simulink model "LAB9PUNKT2"  (R2022b)
settings: Solver=VariableStepAuto  StartTime=0.0  StopTime=10.0  RelTol=1e-3
settings Model: Creator=Wikor  LastModifiedBy=mateu
settings DebuggingCC: UnconnectedInputMsg=warning  UnconnectedOutputMsg=warning  UnconnectedLineMsg=warning
settings ModelReferenceCC: EnableRefExpFcnMdlSchedulingChecks=on
settings RTWCC: DLArmComputeVersion=19.05

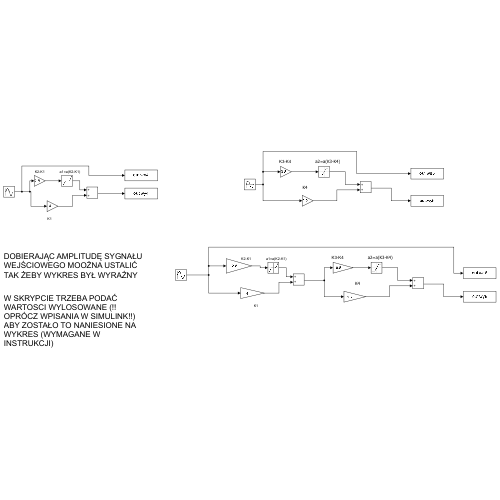
[thumbnail: Simulink's stored preview of the top-level diagram]
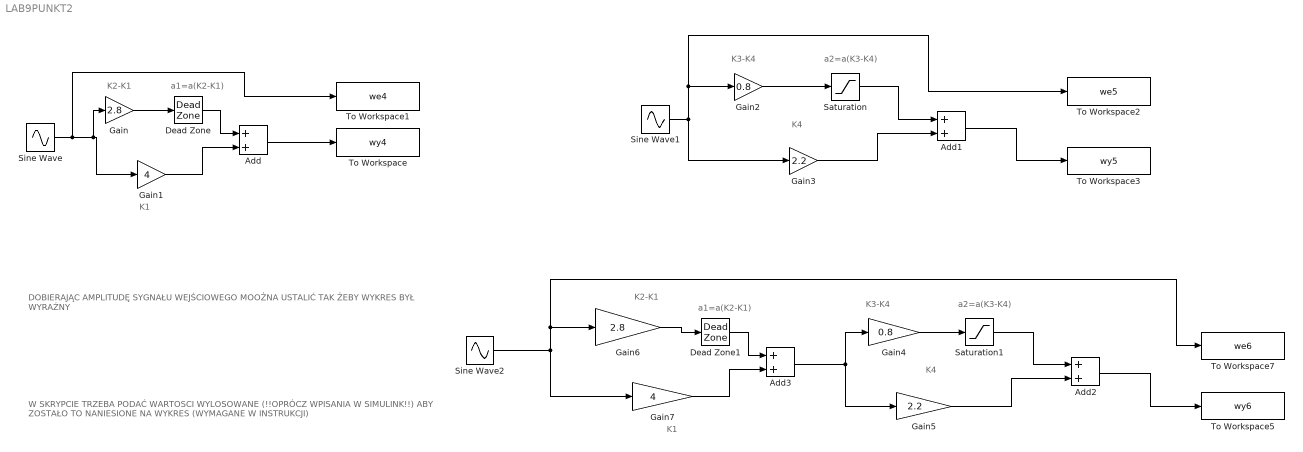
== system LAB9PUNKT2 ==
  note: a2=a(K3-K4)
  note: K3-K4
  note: K4
  note: DOBIERAJĄC AMPLITUDĘ SYGNAŁU WEJŚCIOWEGO MOOŻNA USTALIĆ TAK ŻEBY WYKRES BYŁ WYRAŹNY
  note: K2-K1
  note: a1=a(K2-K1)
  note: K1
  note: W SKRYPCIE TRZEBA PODAĆ WARTOSCI WYLOSOWANE (!!OPRÓCZ WPISANIA W SIMULINK!!) ABY ZOSTAŁO TO NANIESIONE NA WYKRES (WYMAGANE W INSTRUKCJI)
  note: K3-K4
  note: a2=a(K3-K4)
  note: K4
  note: K2-K1
  note: K1
  note: a1=a(K2-K1)
  Add{,1..3} (4 alike) : Sum
  Dead Zone : DeadZone  LowerValue=-3.92  UpperValue=3.92
  Dead Zone1 : DeadZone  LowerValue=-3.92  UpperValue=3.92
  Gain : Gain  Gain=2.8
  Gain1 : Gain  Gain=4
  Gain2 : Gain  Gain=0.8
  Gain3 : Gain  Gain=2.2
  Gain4 : Gain  Gain=0.8
  Gain5 : Gain  Gain=2.2
  Gain6 : Gain  Gain=2.8
  Gain7 : Gain  Gain=4
  Saturation : Saturate  UpperLimit=1.12  LowerLimit=-1.12
  Saturation1 : Saturate  UpperLimit=1.12  LowerLimit=-1.12
  Sine Wave : Sin  Amplitude=4  SampleTime=0
  Sine Wave1 : Sin  Amplitude=5  SampleTime=0
  Sine Wave2 : Sin  Amplitude=15  SampleTime=0
  To Workspace : ToWorkspace  VariableName=wy4  SampleTime=-1
  To Workspace1 : ToWorkspace  VariableName=we4  SampleTime=-1
  To Workspace2 : ToWorkspace  VariableName=we5  SampleTime=-1
  To Workspace3 : ToWorkspace  VariableName=wy5  SampleTime=-1
  To Workspace5 : ToWorkspace  VariableName=wy6  SampleTime=-1
  To Workspace7 : ToWorkspace  VariableName=we6  SampleTime=-1
  wires:
  Add/1 -> To Workspace/1
  Gain1/1 -> Add/2
  Sine Wave/1 -> To Workspace1/1, Gain/1, Gain1/1
  Gain/1 -> Dead Zone/1
  Dead Zone/1 -> Add/1
  Saturation/1 -> Add1/1
  Gain3/1 -> Add1/2
  Add1/1 -> To Workspace3/1
  Sine Wave1/1 -> Gain3/1, To Workspace2/1, Gain2/1
  Gain2/1 -> Saturation/1
  Saturation1/1 -> Add2/1
  Gain5/1 -> Add2/2
  Gain4/1 -> Saturation1/1
  Add2/1 -> To Workspace5/1
  Gain7/1 -> Add3/2
  Dead Zone1/1 -> Add3/1
  Sine Wave2/1 -> Gain6/1, To Workspace7/1, Gain7/1
  Gain6/1 -> Dead Zone1/1
  Add3/1 -> Gain4/1, Gain5/1
